simulink model "IEEE80211a"  (Simulink 10.0)
settings: Solver=FixedStepDiscrete  StartTime=0.0  StopTime=inf  RelTol=1e-3
PreLoadFcn:
  | load IEEE80211a_init;
undefined symbols (not defined in the file): hyst, magnitude, params, QAM, thres
libraries: simulink x27, IEEE80211a_lib x22, dspmtrx3 x15, dspsigops x11, dspsigattribs x9, dspobslib x6, dspstat3 x6, dspmathops x5, dspindex x3, commchan2 x3, dspbuff3 x2, dspxfrm3 x2
(part 2 of 2)

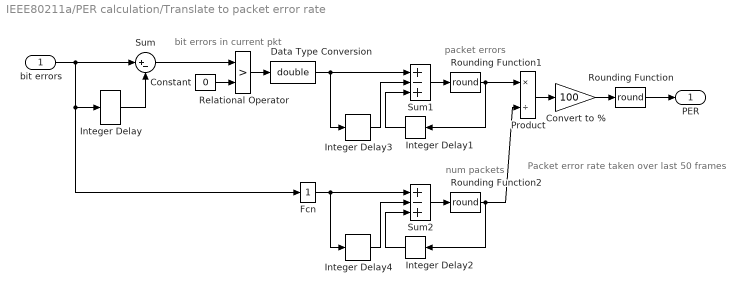
== system IEEE80211a/PER calculation/Translate to packet error rate ==
  note: Packet error rate taken over last 50 frames
  note: bit errors in
      | current pkt
  note: packet errors
  note: num packets
  bit errors : Inport
  Constant : Constant  Value=0
  Convert to % : Gain  Gain=100  SaturateOnIntegerOverflow=on  OutDataTypeStr=Inherit: Same as input  ParamDataTypeStr=Inherit: Same as input
  Data Type Conversion : DataTypeConversion  OutDataTypeStr=double  SaturateOnIntegerOverflow=on  RndMeth=Zero
  Fcn : Fcn  Expr=1
  Integer Delay : dspobslib/Integer Delay  delay=1  ic=0  reset_popup=None
      settings: SourceProductName=DSP System Toolbox  SourceProductBaseCode=DS
  Integer Delay1 : dspobslib/Integer Delay  delay=1  ic=0  reset_popup=None
      settings: SourceProductName=DSP System Toolbox  SourceProductBaseCode=DS
  Integer Delay2 : dspobslib/Integer Delay  delay=1  ic=0  reset_popup=None
      settings: SourceProductName=DSP System Toolbox  SourceProductBaseCode=DS
  Integer Delay3 : dspobslib/Integer Delay  delay=50  ic=0  reset_popup=None
      settings: SourceProductName=DSP System Toolbox  SourceProductBaseCode=DS
  Integer Delay4 : dspobslib/Integer Delay  delay=50  ic=0  reset_popup=None
      settings: SourceProductName=DSP System Toolbox  SourceProductBaseCode=DS
  Product : Product  Inputs=*/  SaturateOnIntegerOverflow=on  OutDataTypeStr=Inherit: Same as first input
  Relational Operator : RelationalOperator  Operator=>  RndMeth=Nearest
  Rounding Function : Rounding  Operator=round
  Rounding Function1 : Rounding  Operator=round
  Rounding Function2 : Rounding  Operator=round
  Sum : Sum  Inputs=|+-  SaturateOnIntegerOverflow=on
  Sum1 : Sum  Inputs=+-+  SaturateOnIntegerOverflow=on
  Sum2 : Sum  Inputs=+-+  SaturateOnIntegerOverflow=on
  PER : Outport
  wires:
  Rounding Function2/1 -> Integer Delay2/1, Product/2
  Rounding Function1/1 -> Integer Delay1/1, Product/1
  Rounding Function/1 -> PER/1
  Sum1/1 -> Rounding Function1/1
  Integer Delay1/1 -> Sum1/3
  Integer Delay3/1 -> Sum1/2
  Data Type Conversion/1 -> Sum1/1, Integer Delay3/1
  Integer Delay2/1 -> Sum2/3
  Integer Delay4/1 -> Sum2/2
  Sum2/1 -> Rounding Function2/1
  bit errors/1 -> Fcn/1, Integer Delay/1, Sum/1
  Convert to %/1 -> Rounding Function/1
  Product/1 -> Convert to %/1
  Fcn/1 -> Integer Delay4/1, Sum2/1
  Constant/1 -> Relational Operator/2
  Relational Operator/1 -> Data Type Conversion/1
  Sum/1 -> Relational Operator/1
  Integer Delay/1 -> Sum/2
